simulink model "trenl"  (Simulink 10.2)
settings: Solver=ode45  StartTime=0.0  StopTime=Time  RelTol=1e-3  EnableMultiTasking=on
values from neighbouring files (symbols this model uses):
  n = 10    [lab3var4.m]
undefined symbols (not defined in the file or in its folder): m
settings Model: Creator=mitrofanova  LastModifiedBy=gorbushin_v_a
settings DataIOCC: LimitDataPoints=on  SignalLoggingName=sigsOut
settings OptimizationCC: ExpressionDepthLimit=2147483647  InitFltsAndDblsToZero=on
settings DebuggingCC: SaveWithParameterizedLinksMsg=none  SignalResolutionControl=TryResolveAllWithWarning  MultiTaskDSMMsg=warning  MultiTaskCondExecSysMsg=none  StateNameClashWarn=warning
settings HardwareCC: TargetUnknown=on
settings GRTTargetCC: TargetFcnLib=ansi_tfl_tmw.mat

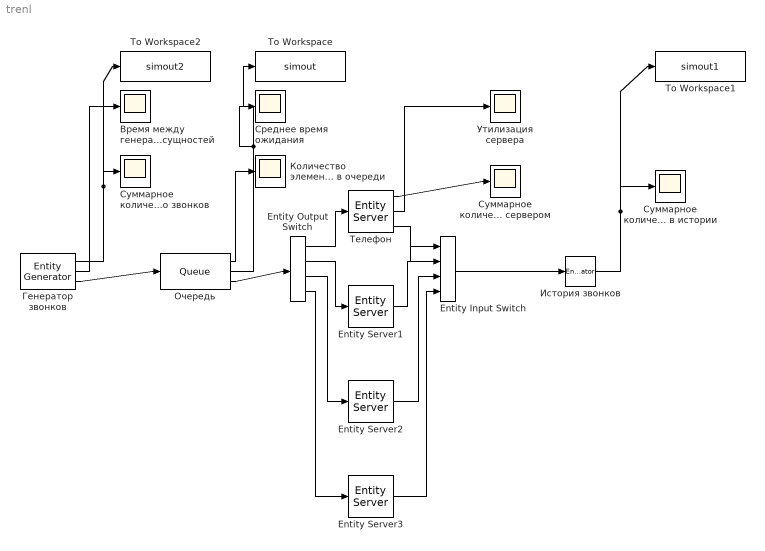
== system trenl ==
  Entity Input Switch : EntityInputSwitch  InputPortMessageModes=m,m,m,m  OutputPortMessageModes=m  NumberInputPorts=4
      settings: InputPortMap=u1,u2,u3,u4
  Entity Output Switch : EntityOutputSwitch  InputPortMessageModes=m  OutputPortMessageModes=m,m,m,m  NumberOutputPorts=4  SwitchAttributeName=Attribute1
      settings: OutputPortMap=o0,o1,o2,o3
  Entity Server1 : EntityServer  InputPortMessageModes=m  OutputPortMessageModes=m  Capacity=1  ServiceTimeValue=ServiceTime
  Entity Server2 : EntityServer  InputPortMessageModes=m  OutputPortMessageModes=m  Capacity=1  ServiceTimeValue=ServiceTime
  Entity Server3 : EntityServer  InputPortMessageModes=m  OutputPortMessageModes=m  Capacity=1  ServiceTimeValue=ServiceTime
  To Workspace : ToWorkspace  VariableName=simout  SampleTime=-1
  To Workspace1 : ToWorkspace  VariableName=simout1  SampleTime=-1
  To Workspace2 : ToWorkspace  VariableName=simout2  SampleTime=-1
  Время между генерациями сущностей : Scope
  Генератор звонков : EntityGenerator  OutputPortMessageModes=n,n,m  TimeSource=MATLAB action  IntergenerationTimeAction=dt = exprnd(1/25);  NumberEntitiesDeparted=on  AverageIntergenerationTime=on  EntityType=Structured  EntityTypeName=Entity
      settings: OutputPortMap=o0,o2,o3
  История звонков : EntityTerminator  InputPortMessageModes=m  NumberEntitiesArrived=on
      settings: OutputPortMap=o0
  Количество  элементов в очереди : Scope
  Очередь : Queue  InputPortMessageModes=m  OutputPortMessageModes=n,n,m  Capacity=QueueCapacity  NumberEntitiesInBlock=on  AverageWait=on
      settings: OutputPortMap=o1,o2,o5
  Среднее время ожидания : Scope
  "Суммарное количесиво звонков, обработанных 1 сервером" : Scope
  Суммарное количество звонков : Scope
  Суммарное количество звонков в истории : Scope
  Телефон : EntityServer  InputPortMessageModes=m  OutputPortMessageModes=n,n,m  Capacity=1  ServiceTimeValue=ServiceTime  NumberEntitiesDeparted=on  Utilization=on
      settings: OutputPortMap=o0,o5,o9
  Утилизация сервера : Scope
  wires:
  Генератор звонков/3 -> Очередь/1
  Очередь/2 -> To Workspace/1, Среднее время ожидания/1
  История звонков/1 -> To Workspace1/1, Суммарное количество звонков в истории/1
  Генератор звонков/2 -> Время между генерациями сущностей/1
  Генератор звонков/1 -> To Workspace2/1, Суммарное количество звонков/1
  Телефон/2 -> Утилизация сервера/1
  Очередь/3 -> Entity Output Switch/1
  Entity Output Switch/1 -> Телефон/1
  Entity Input Switch/1 -> История звонков/1
  Entity Output Switch/2 -> Entity Server1/1
  Телефон/3 -> Entity Input Switch/1
  Entity Server1/1 -> Entity Input Switch/2
  Entity Output Switch/3 -> Entity Server2/1
  Entity Output Switch/4 -> Entity Server3/1
  Entity Server2/1 -> Entity Input Switch/3
  Entity Server3/1 -> Entity Input Switch/4
  Телефон/1 -> "Суммарное количесиво звонков, обработанных 1 сервером"/1
  Очередь/1 -> Количество  элементов в очереди/1
